simulink model "helicopter"  (R2021a)
settings: Solver=VariableStepAuto  StartTime=0.0  StopTime=10  RelTol=1e-3
values from neighbouring files (symbols this model uses):
  A = [-0.4 0 -0.01; 1 0 0; -1.4 9.8 -0.02]    [exc4.m]
  B = [6.3; 0; 9.8]    [exc4.m]
  C = eye(3)    [exc4.m]
  D = [0; 0; 0]    [exc4.m]
  K = place(A, B, [-1 -5 -10])    [exc4.m]
undefined symbols (not defined in the file or in its folder): K_lqr, K_lqr_d
settings Model: Creator=davidrico  LastModifiedBy=davidrico

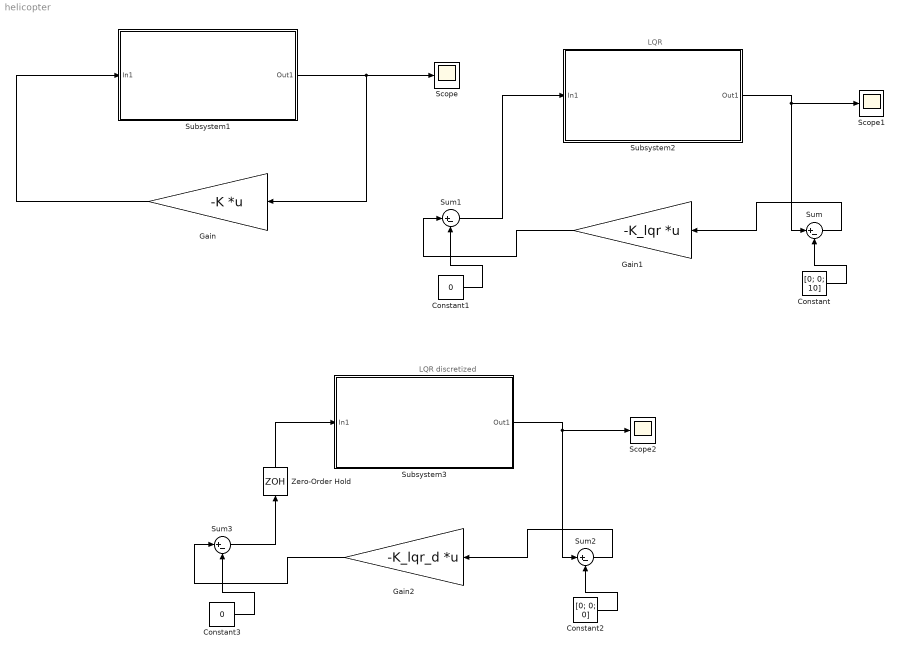
== system helicopter ==
  note: LQR
  note: LQR discretized
  Constant : Constant  Value=[0; 0; 10]
  Constant1 : Constant  Value=0
  Constant2 : Constant  Value=[0; 0; 0]
  Constant3 : Constant  Value=0
  Gain : Gain  Gain=-K  Multiplication=Matrix(K*u) (u vector)
  Gain1 : Gain  Gain=-K_lqr  Multiplication=Matrix(K*u) (u vector)
  Gain2 : Gain  Gain=-K_lqr_d  Multiplication=Matrix(K*u) (u vector)
  Scope : Scope
  Scope1 : Scope
  Scope2 : Scope
  Subsystem1 : Subsystem
  Subsystem2 : Subsystem
  Subsystem3 : Subsystem
  Sum{,1..3} (4 alike) : Sum  Inputs=|+-
  Zero-Order Hold : ZeroOrderHold  SampleTime=10
  wires:
  Subsystem1/1(Out1) -> Gain/1, Scope/1
  Gain/1 -> Subsystem1/1(In1)
  Subsystem2/1(Out1) -> Sum/1, Scope1/1
  Sum/1 -> Gain1/1
  Constant/1 -> Sum/2
  Gain1/1 -> Sum1/1
  Sum1/1 -> Subsystem2/1(In1)
  Constant1/1 -> Sum1/2
  Gain2/1 -> Sum3/1
  Constant2/1 -> Sum2/2
  Sum2/1 -> Gain2/1
  Subsystem3/1(Out1) -> Sum2/1, Scope2/1
  Sum3/1 -> Zero-Order Hold/1
  Constant3/1 -> Sum3/2
  Zero-Order Hold/1 -> Subsystem3/1(In1)

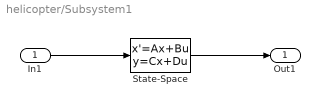
== system helicopter/Subsystem1 ==
  In1 : Inport
  State-Space : StateSpace  A=A  B=B  C=C  D=D  InitialCondition=[1; 1; 1]
  Out1 : Outport
  wires:
  In1/1 -> State-Space/1
  State-Space/1 -> Out1/1

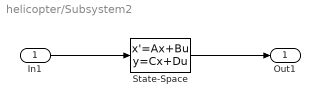
== system helicopter/Subsystem2 ==
  In1 : Inport
  State-Space : StateSpace  A=A  B=B  C=C  D=D  InitialCondition=[1; 1; 1]
  Out1 : Outport
  wires:
  In1/1 -> State-Space/1
  State-Space/1 -> Out1/1

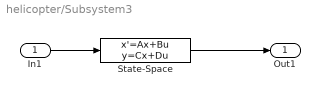
== system helicopter/Subsystem3 ==
  In1 : Inport
  State-Space : StateSpace  A=A  B=B  C=C  D=D  InitialCondition=[1; 1; 1]
  Out1 : Outport
  wires:
  In1/1 -> State-Space/1
  State-Space/1 -> Out1/1
